simulink model "testing"  (R2013b)
settings: Solver=ode45  StartTime=0.0  StopTime=10.0  RelTol=1e-3
undefined symbols (not defined in the file or in its folder): xlfda_numerator, xlipgetpartsetting
libraries: xbsIndex_r4 x1880, casper_library_delays x19, dspsigops x16, casper_library_misc x8, simulink x1, xps_library x1
(part 10 of 17)

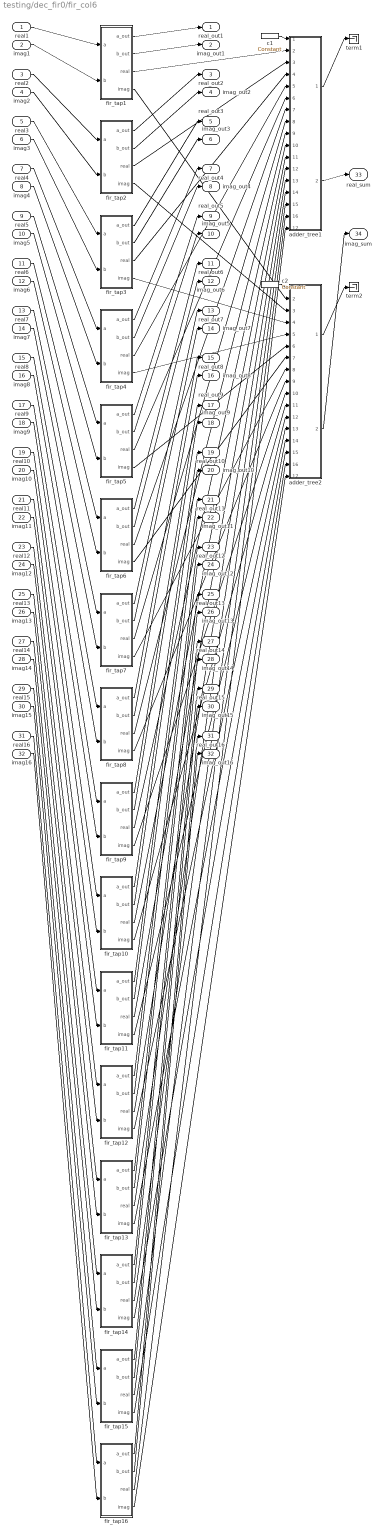
== system testing/dec_fir0/fir_col6 ==
  real1 : Inport
  imag1 : Inport  Port=2
  real2 : Inport  Port=3
  imag2 : Inport  Port=4
  real3 : Inport  Port=5
  imag3 : Inport  Port=6
  real4 : Inport  Port=7
  imag4 : Inport  Port=8
  real5 : Inport  Port=9
  imag5 : Inport  Port=10
  real6 : Inport  Port=11
  imag6 : Inport  Port=12
  real7 : Inport  Port=13
  imag7 : Inport  Port=14
  real8 : Inport  Port=15
  imag8 : Inport  Port=16
  real9 : Inport  Port=17
  imag9 : Inport  Port=18
  real10 : Inport  Port=19
  imag10 : Inport  Port=20
  real11 : Inport  Port=21
  imag11 : Inport  Port=22
  real12 : Inport  Port=23
  imag12 : Inport  Port=24
  real13 : Inport  Port=25
  imag13 : Inport  Port=26
  real14 : Inport  Port=27
  imag14 : Inport  Port=28
  real15 : Inport  Port=29
  imag15 : Inport  Port=30
  real16 : Inport  Port=31
  imag16 : Inport  Port=32
  adder_tree1 : Subsystem  AncestorBlock=casper_library_misc/adder_tree  mask(adder_tree){n_inputs=16, latency=1, adder_imp=DSP48, first_stage_hdl=on}
      mask prompts: n_inputs "Number of Inputs"; latency "Add Latency"; adder_imp "Adder implementation"; first_stage_hdl "Use behavioural HDL for first stage of adders"
      mask help:
      | Sums all inputs using a tree of adds and delays.
      |
      | Number of inputs: The number of inputs to the block to be summed
      | Add latency: The number of clock cycles to perform one addition (affects timing)..
      | Adder implementation: choice of fabric or DSP48E core, or behavioral HDL
      | Use behavioural HDL for first stage of adders: Causes the first stage of adders to be absorbed into DSP blocks if multipliers precede them (Virtex 5). Overrides Adder implementation
      mask init:
      | adder_tree_init(gcb, ...
      |     'n_inputs', n_inputs, ...
      |     'latency', latency, ...
      |     'adder_imp', adder_imp, ...
      |     'first_stage_hdl', first_stage_hdl);
      settings: AttributesFormatString=latency 4
      mask Help: eval('xlWeb(''http://casper.berkeley.edu/wiki/Adder_tree'')')
      mask TypeOptions adder_imp: Behavioral | Fabric | DSP48
  adder_tree2 : Subsystem  AncestorBlock=casper_library_misc/adder_tree  mask(adder_tree){n_inputs=16, latency=1, adder_imp=DSP48, first_stage_hdl=on}
      mask prompts: n_inputs "Number of Inputs"; latency "Add Latency"; adder_imp "Adder implementation"; first_stage_hdl "Use behavioural HDL for first stage of adders"
      mask help:
      | Sums all inputs using a tree of adds and delays.
      |
      | Number of inputs: The number of inputs to the block to be summed
      | Add latency: The number of clock cycles to perform one addition (affects timing)..
      | Adder implementation: choice of fabric or DSP48E core, or behavioral HDL
      | Use behavioural HDL for first stage of adders: Causes the first stage of adders to be absorbed into DSP blocks if multipliers precede them (Virtex 5). Overrides Adder implementation
      mask init:
      | adder_tree_init(gcb, ...
      |     'n_inputs', n_inputs, ...
      |     'latency', latency, ...
      |     'adder_imp', adder_imp, ...
      |     'first_stage_hdl', first_stage_hdl);
      settings: AttributesFormatString=latency 4
      mask Help: eval('xlWeb(''http://casper.berkeley.edu/wiki/Adder_tree'')')
      mask TypeOptions adder_imp: Behavioral | Fabric | DSP48
  c1 : xbsIndex_r4/Constant  const=1  gui_display_data_type=Fixed-point  arith_type=Signed (2's comp)  n_bits=16  bin_pt=14  preci_type=Single  exp_width=8  frac_width=24  explicit_period=on  period=1  equ=P=C  opselect=C  inp2=PCIN>>17  opr=+  inp1=P  carry=CIN  dbl_ovrd=off  block_type=constant
  c2 : xbsIndex_r4/Constant  const=1  gui_display_data_type=Fixed-point  arith_type=Signed (2's comp)  n_bits=16  bin_pt=14  preci_type=Single  exp_width=8  frac_width=24  explicit_period=on  period=1  equ=P=C  opselect=C  inp2=PCIN>>17  opr=+  inp1=P  carry=CIN  dbl_ovrd=off  block_type=constant
  fir_tap1 : Subsystem  AncestorBlock=casper_library_downconverter/fir_tap  mask(fir_tap){factor=0.0068851, latency=2, coeff_bit_width=25, coeff_bin_pt=24}
      mask prompts: latency "Mult latency"; coeff_bit_width "Coefficient bit width"; coeff_bin_pt "Coefficient binary point"
      mask help: Multiplies input data with factor specified.
      mask init:
      | fir_tap_init(gcb, ...
      |     'factor', factor, ...
      |     'latency', latency, ...
      |     'coeff_bit_width', coeff_bit_width, ...
      |     'coeff_bin_pt', coeff_bin_pt);
      mask Help: eval('xlWeb(''http://casper.berkeley.edu/wiki/Fir_tap'')')
  fir_tap10 : Subsystem  AncestorBlock=casper_library_downconverter/fir_tap  mask(fir_tap){factor=-0.00040564, latency=2, coeff_bit_width=25, coeff_bin_pt=24}
      mask prompts: latency "Mult latency"; coeff_bit_width "Coefficient bit width"; coeff_bin_pt "Coefficient binary point"
      mask help: Multiplies input data with factor specified.
      mask init:
      | fir_tap_init(gcb, ...
      |     'factor', factor, ...
      |     'latency', latency, ...
      |     'coeff_bit_width', coeff_bit_width, ...
      |     'coeff_bin_pt', coeff_bin_pt);
      mask Help: eval('xlWeb(''http://casper.berkeley.edu/wiki/Fir_tap'')')
  fir_tap11 : Subsystem  AncestorBlock=casper_library_downconverter/fir_tap  mask(fir_tap){factor=-0.002452, latency=2, coeff_bit_width=25, coeff_bin_pt=24}
      mask prompts: latency "Mult latency"; coeff_bit_width "Coefficient bit width"; coeff_bin_pt "Coefficient binary point"
      mask help: Multiplies input data with factor specified.
      mask init:
      | fir_tap_init(gcb, ...
      |     'factor', factor, ...
      |     'latency', latency, ...
      |     'coeff_bit_width', coeff_bit_width, ...
      |     'coeff_bin_pt', coeff_bin_pt);
      mask Help: eval('xlWeb(''http://casper.berkeley.edu/wiki/Fir_tap'')')
  fir_tap12 : Subsystem  AncestorBlock=casper_library_downconverter/fir_tap  mask(fir_tap){factor=-0.0045559, latency=2, coeff_bit_width=25, coeff_bin_pt=24}
      mask prompts: latency "Mult latency"; coeff_bit_width "Coefficient bit width"; coeff_bin_pt "Coefficient binary point"
      mask help: Multiplies input data with factor specified.
      mask init:
      | fir_tap_init(gcb, ...
      |     'factor', factor, ...
      |     'latency', latency, ...
      |     'coeff_bit_width', coeff_bit_width, ...
      |     'coeff_bin_pt', coeff_bin_pt);
      mask Help: eval('xlWeb(''http://casper.berkeley.edu/wiki/Fir_tap'')')
  fir_tap13 : Subsystem  AncestorBlock=casper_library_downconverter/fir_tap  mask(fir_tap){factor=-0.0066339, latency=2, coeff_bit_width=25, coeff_bin_pt=24}
      mask prompts: latency "Mult latency"; coeff_bit_width "Coefficient bit width"; coeff_bin_pt "Coefficient binary point"
      mask help: Multiplies input data with factor specified.
      mask init:
      | fir_tap_init(gcb, ...
      |     'factor', factor, ...
      |     'latency', latency, ...
      |     'coeff_bit_width', coeff_bit_width, ...
      |     'coeff_bin_pt', coeff_bin_pt);
      mask Help: eval('xlWeb(''http://casper.berkeley.edu/wiki/Fir_tap'')')
  fir_tap14 : Subsystem  AncestorBlock=casper_library_downconverter/fir_tap  mask(fir_tap){factor=-0.0085971, latency=2, coeff_bit_width=25, coeff_bin_pt=24}
      mask prompts: latency "Mult latency"; coeff_bit_width "Coefficient bit width"; coeff_bin_pt "Coefficient binary point"
      mask help: Multiplies input data with factor specified.
      mask init:
      | fir_tap_init(gcb, ...
      |     'factor', factor, ...
      |     'latency', latency, ...
      |     'coeff_bit_width', coeff_bit_width, ...
      |     'coeff_bin_pt', coeff_bin_pt);
      mask Help: eval('xlWeb(''http://casper.berkeley.edu/wiki/Fir_tap'')')
  fir_tap15 : Subsystem  AncestorBlock=casper_library_downconverter/fir_tap  mask(fir_tap){factor=-0.010354, latency=2, coeff_bit_width=25, coeff_bin_pt=24}
      mask prompts: latency "Mult latency"; coeff_bit_width "Coefficient bit width"; coeff_bin_pt "Coefficient binary point"
      mask help: Multiplies input data with factor specified.
      mask init:
      | fir_tap_init(gcb, ...
      |     'factor', factor, ...
      |     'latency', latency, ...
      |     'coeff_bit_width', coeff_bit_width, ...
      |     'coeff_bin_pt', coeff_bin_pt);
      mask Help: eval('xlWeb(''http://casper.berkeley.edu/wiki/Fir_tap'')')
  fir_tap16 : Subsystem  AncestorBlock=casper_library_downconverter/fir_tap  mask(fir_tap){factor=-0.011813, latency=2, coeff_bit_width=25, coeff_bin_pt=24}
      mask prompts: latency "Mult latency"; coeff_bit_width "Coefficient bit width"; coeff_bin_pt "Coefficient binary point"
      mask help: Multiplies input data with factor specified.
      mask init:
      | fir_tap_init(gcb, ...
      |     'factor', factor, ...
      |     'latency', latency, ...
      |     'coeff_bit_width', coeff_bit_width, ...
      |     'coeff_bin_pt', coeff_bin_pt);
      mask Help: eval('xlWeb(''http://casper.berkeley.edu/wiki/Fir_tap'')')
  fir_tap2 : Subsystem  AncestorBlock=casper_library_downconverter/fir_tap  mask(fir_tap){factor=0.007301, latency=2, coeff_bit_width=25, coeff_bin_pt=24}
      mask prompts: latency "Mult latency"; coeff_bit_width "Coefficient bit width"; coeff_bin_pt "Coefficient binary point"
      mask help: Multiplies input data with factor specified.
      mask init:
      | fir_tap_init(gcb, ...
      |     'factor', factor, ...
      |     'latency', latency, ...
      |     'coeff_bit_width', coeff_bit_width, ...
      |     'coeff_bin_pt', coeff_bin_pt);
      mask Help: eval('xlWeb(''http://casper.berkeley.edu/wiki/Fir_tap'')')
  fir_tap3 : Subsystem  AncestorBlock=casper_library_downconverter/fir_tap  mask(fir_tap){factor=0.0074255, latency=2, coeff_bit_width=25, coeff_bin_pt=24}
      mask prompts: latency "Mult latency"; coeff_bit_width "Coefficient bit width"; coeff_bin_pt "Coefficient binary point"
      mask help: Multiplies input data with factor specified.
      mask init:
      | fir_tap_init(gcb, ...
      |     'factor', factor, ...
      |     'latency', latency, ...
      |     'coeff_bit_width', coeff_bit_width, ...
      |     'coeff_bin_pt', coeff_bin_pt);
      mask Help: eval('xlWeb(''http://casper.berkeley.edu/wiki/Fir_tap'')')
  fir_tap4 : Subsystem  AncestorBlock=casper_library_downconverter/fir_tap  mask(fir_tap){factor=0.0072334, latency=2, coeff_bit_width=25, coeff_bin_pt=24}
      mask prompts: latency "Mult latency"; coeff_bit_width "Coefficient bit width"; coeff_bin_pt "Coefficient binary point"
      mask help: Multiplies input data with factor specified.
      mask init:
      | fir_tap_init(gcb, ...
      |     'factor', factor, ...
      |     'latency', latency, ...
      |     'coeff_bit_width', coeff_bit_width, ...
      |     'coeff_bin_pt', coeff_bin_pt);
      mask Help: eval('xlWeb(''http://casper.berkeley.edu/wiki/Fir_tap'')')
  fir_tap5 : Subsystem  AncestorBlock=casper_library_downconverter/fir_tap  mask(fir_tap){factor=0.0067112, latency=2, coeff_bit_width=25, coeff_bin_pt=24}
      mask prompts: latency "Mult latency"; coeff_bit_width "Coefficient bit width"; coeff_bin_pt "Coefficient binary point"
      mask help: Multiplies input data with factor specified.
      mask init:
      | fir_tap_init(gcb, ...
      |     'factor', factor, ...
      |     'latency', latency, ...
      |     'coeff_bit_width', coeff_bit_width, ...
      |     'coeff_bin_pt', coeff_bin_pt);
      mask Help: eval('xlWeb(''http://casper.berkeley.edu/wiki/Fir_tap'')')
  fir_tap6 : Subsystem  AncestorBlock=casper_library_downconverter/fir_tap  mask(fir_tap){factor=0.005858, latency=2, coeff_bit_width=25, coeff_bin_pt=24}
      mask prompts: latency "Mult latency"; coeff_bit_width "Coefficient bit width"; coeff_bin_pt "Coefficient binary point"
      mask help: Multiplies input data with factor specified.
      mask init:
      | fir_tap_init(gcb, ...
      |     'factor', factor, ...
      |     'latency', latency, ...
      |     'coeff_bit_width', coeff_bit_width, ...
      |     'coeff_bin_pt', coeff_bin_pt);
      mask Help: eval('xlWeb(''http://casper.berkeley.edu/wiki/Fir_tap'')')
  fir_tap7 : Subsystem  AncestorBlock=casper_library_downconverter/fir_tap  mask(fir_tap){factor=0.0046863, latency=2, coeff_bit_width=25, coeff_bin_pt=24}
      mask prompts: latency "Mult latency"; coeff_bit_width "Coefficient bit width"; coeff_bin_pt "Coefficient binary point"
      mask help: Multiplies input data with factor specified.
      mask init:
      | fir_tap_init(gcb, ...
      |     'factor', factor, ...
      |     'latency', latency, ...
      |     'coeff_bit_width', coeff_bit_width, ...
      |     'coeff_bin_pt', coeff_bin_pt);
      mask Help: eval('xlWeb(''http://casper.berkeley.edu/wiki/Fir_tap'')')
  fir_tap8 : Subsystem  AncestorBlock=casper_library_downconverter/fir_tap  mask(fir_tap){factor=0.0032228, latency=2, coeff_bit_width=25, coeff_bin_pt=24}
      mask prompts: latency "Mult latency"; coeff_bit_width "Coefficient bit width"; coeff_bin_pt "Coefficient binary point"
      mask help: Multiplies input data with factor specified.
      mask init:
      | fir_tap_init(gcb, ...
      |     'factor', factor, ...
      |     'latency', latency, ...
      |     'coeff_bit_width', coeff_bit_width, ...
      |     'coeff_bin_pt', coeff_bin_pt);
      mask Help: eval('xlWeb(''http://casper.berkeley.edu/wiki/Fir_tap'')')
  fir_tap9 : Subsystem  AncestorBlock=casper_library_downconverter/fir_tap  mask(fir_tap){factor=0.0015077, latency=2, coeff_bit_width=25, coeff_bin_pt=24}
      mask prompts: latency "Mult latency"; coeff_bit_width "Coefficient bit width"; coeff_bin_pt "Coefficient binary point"
      mask help: Multiplies input data with factor specified.
      mask init:
      | fir_tap_init(gcb, ...
      |     'factor', factor, ...
      |     'latency', latency, ...
      |     'coeff_bit_width', coeff_bit_width, ...
      |     'coeff_bin_pt', coeff_bin_pt);
      mask Help: eval('xlWeb(''http://casper.berkeley.edu/wiki/Fir_tap'')')
  term1 : Terminator
  term2 : Terminator
  real_out1 : Outport
  imag_out1 : Outport  Port=2
  real_out2 : Outport  Port=3
  imag_out2 : Outport  Port=4
  real_out3 : Outport  Port=5
  imag_out3 : Outport  Port=6
  real_out4 : Outport  Port=7
  imag_out4 : Outport  Port=8
  real_out5 : Outport  Port=9
  imag_out5 : Outport  Port=10
  real_out6 : Outport  Port=11
  imag_out6 : Outport  Port=12
  real_out7 : Outport  Port=13
  imag_out7 : Outport  Port=14
  real_out8 : Outport  Port=15
  imag_out8 : Outport  Port=16
  real_out9 : Outport  Port=17
  imag_out9 : Outport  Port=18
  real_out10 : Outport  Port=19
  imag_out10 : Outport  Port=20
  real_out11 : Outport  Port=21
  imag_out11 : Outport  Port=22
  real_out12 : Outport  Port=23
  imag_out12 : Outport  Port=24
  real_out13 : Outport  Port=25
  imag_out13 : Outport  Port=26
  real_out14 : Outport  Port=27
  imag_out14 : Outport  Port=28
  real_out15 : Outport  Port=29
  imag_out15 : Outport  Port=30
  real_out16 : Outport  Port=31
  imag_out16 : Outport  Port=32
  real_sum : Outport  Port=33
  imag_sum : Outport  Port=34
  wires:
  adder_tree1/1(sync_out) -> term1/1
  adder_tree2/1(sync_out) -> term2/1
  c1/1 -> adder_tree1/1(sync)
  c2/1 -> adder_tree2/1(sync)
  adder_tree1/2(dout) -> real_sum/1
  adder_tree2/2(dout) -> imag_sum/1
  real1/1 -> fir_tap1/1(a)
  imag1/1 -> fir_tap1/2(b)
  fir_tap1/1(a_out) -> real_out1/1
  fir_tap1/2(b_out) -> imag_out1/1
  fir_tap1/3(real) -> adder_tree1/2(din1)
  fir_tap1/4(imag) -> adder_tree2/2(din1)
  real2/1 -> fir_tap2/1(a)
  imag2/1 -> fir_tap2/2(b)
  fir_tap2/1(a_out) -> real_out2/1
  fir_tap2/2(b_out) -> imag_out2/1
  fir_tap2/3(real) -> adder_tree1/3(din2)
  fir_tap2/4(imag) -> adder_tree2/3(din2)
  real3/1 -> fir_tap3/1(a)
  imag3/1 -> fir_tap3/2(b)
  fir_tap3/1(a_out) -> real_out3/1
  fir_tap3/2(b_out) -> imag_out3/1
  fir_tap3/3(real) -> adder_tree1/4(din3)
  fir_tap3/4(imag) -> adder_tree2/4(din3)
  real4/1 -> fir_tap4/1(a)
  imag4/1 -> fir_tap4/2(b)
  fir_tap4/1(a_out) -> real_out4/1
  fir_tap4/2(b_out) -> imag_out4/1
  fir_tap4/3(real) -> adder_tree1/5(din4)
  fir_tap4/4(imag) -> adder_tree2/5(din4)
  real5/1 -> fir_tap5/1(a)
  imag5/1 -> fir_tap5/2(b)
  fir_tap5/1(a_out) -> real_out5/1
  fir_tap5/2(b_out) -> imag_out5/1
  fir_tap5/3(real) -> adder_tree1/6(din5)
  fir_tap5/4(imag) -> adder_tree2/6(din5)
  real6/1 -> fir_tap6/1(a)
  imag6/1 -> fir_tap6/2(b)
  fir_tap6/1(a_out) -> real_out6/1
  fir_tap6/2(b_out) -> imag_out6/1
  fir_tap6/3(real) -> adder_tree1/7(din6)
  fir_tap6/4(imag) -> adder_tree2/7(din6)
  real7/1 -> fir_tap7/1(a)
  imag7/1 -> fir_tap7/2(b)
  fir_tap7/1(a_out) -> real_out7/1
  fir_tap7/2(b_out) -> imag_out7/1
  fir_tap7/3(real) -> adder_tree1/8(din7)
  fir_tap7/4(imag) -> adder_tree2/8(din7)
  real8/1 -> fir_tap8/1(a)
  imag8/1 -> fir_tap8/2(b)
  fir_tap8/1(a_out) -> real_out8/1
  fir_tap8/2(b_out) -> imag_out8/1
  fir_tap8/3(real) -> adder_tree1/9(din8)
  fir_tap8/4(imag) -> adder_tree2/9(din8)
  real9/1 -> fir_tap9/1(a)
  imag9/1 -> fir_tap9/2(b)
  fir_tap9/1(a_out) -> real_out9/1
  fir_tap9/2(b_out) -> imag_out9/1
  fir_tap9/3(real) -> adder_tree1/10(din9)
  fir_tap9/4(imag) -> adder_tree2/10(din9)
  real10/1 -> fir_tap10/1(a)
  imag10/1 -> fir_tap10/2(b)
  fir_tap10/1(a_out) -> real_out10/1
  fir_tap10/2(b_out) -> imag_out10/1
  fir_tap10/3(real) -> adder_tree1/11(din10)
  fir_tap10/4(imag) -> adder_tree2/11(din10)
  real11/1 -> fir_tap11/1(a)
  imag11/1 -> fir_tap11/2(b)
  fir_tap11/1(a_out) -> real_out11/1
  fir_tap11/2(b_out) -> imag_out11/1
  fir_tap11/3(real) -> adder_tree1/12(din11)
  fir_tap11/4(imag) -> adder_tree2/12(din11)
  real12/1 -> fir_tap12/1(a)
  imag12/1 -> fir_tap12/2(b)
  fir_tap12/1(a_out) -> real_out12/1
  fir_tap12/2(b_out) -> imag_out12/1
  fir_tap12/3(real) -> adder_tree1/13(din12)
  fir_tap12/4(imag) -> adder_tree2/13(din12)
  real13/1 -> fir_tap13/1(a)
  imag13/1 -> fir_tap13/2(b)
  fir_tap13/1(a_out) -> real_out13/1
  fir_tap13/2(b_out) -> imag_out13/1
  fir_tap13/3(real) -> adder_tree1/14(din13)
  fir_tap13/4(imag) -> adder_tree2/14(din13)
  real14/1 -> fir_tap14/1(a)
  imag14/1 -> fir_tap14/2(b)
  fir_tap14/1(a_out) -> real_out14/1
  fir_tap14/2(b_out) -> imag_out14/1
  fir_tap14/3(real) -> adder_tree1/15(din14)
  fir_tap14/4(imag) -> adder_tree2/15(din14)
  real15/1 -> fir_tap15/1(a)
  imag15/1 -> fir_tap15/2(b)
  fir_tap15/1(a_out) -> real_out15/1
  fir_tap15/2(b_out) -> imag_out15/1
  fir_tap15/3(real) -> adder_tree1/16(din15)
  fir_tap15/4(imag) -> adder_tree2/16(din15)
  real16/1 -> fir_tap16/1(a)
  imag16/1 -> fir_tap16/2(b)
  fir_tap16/1(a_out) -> real_out16/1
  fir_tap16/2(b_out) -> imag_out16/1
  fir_tap16/3(real) -> adder_tree1/17(din16)
  fir_tap16/4(imag) -> adder_tree2/17(din16)

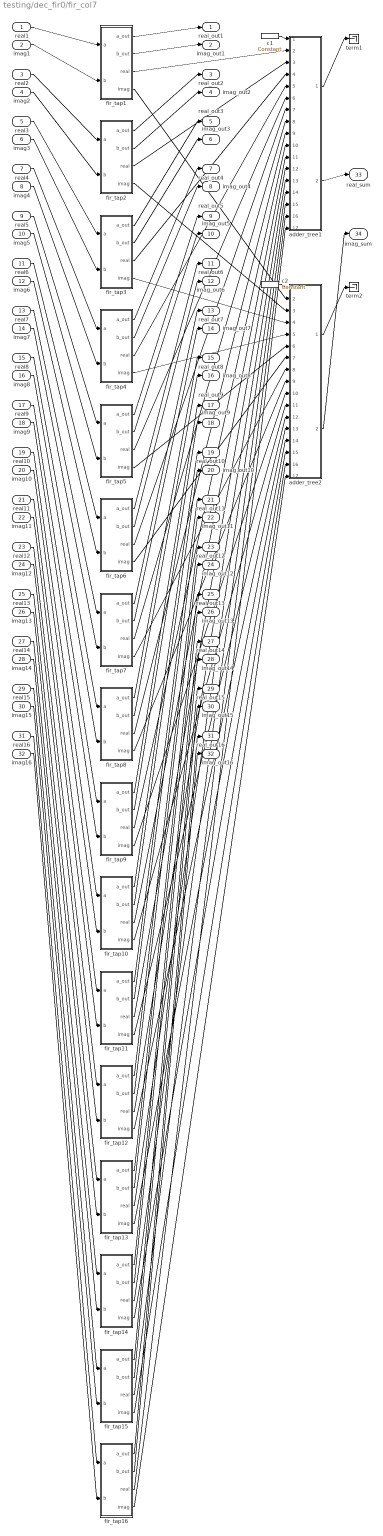
== system testing/dec_fir0/fir_col7 ==
  real1 : Inport
  imag1 : Inport  Port=2
  real2 : Inport  Port=3
  imag2 : Inport  Port=4
  real3 : Inport  Port=5
  imag3 : Inport  Port=6
  real4 : Inport  Port=7
  imag4 : Inport  Port=8
  real5 : Inport  Port=9
  imag5 : Inport  Port=10
  real6 : Inport  Port=11
  imag6 : Inport  Port=12
  real7 : Inport  Port=13
  imag7 : Inport  Port=14
  real8 : Inport  Port=15
  imag8 : Inport  Port=16
  real9 : Inport  Port=17
  imag9 : Inport  Port=18
  real10 : Inport  Port=19
  imag10 : Inport  Port=20
  real11 : Inport  Port=21
  imag11 : Inport  Port=22
  real12 : Inport  Port=23
  imag12 : Inport  Port=24
  real13 : Inport  Port=25
  imag13 : Inport  Port=26
  real14 : Inport  Port=27
  imag14 : Inport  Port=28
  real15 : Inport  Port=29
  imag15 : Inport  Port=30
  real16 : Inport  Port=31
  imag16 : Inport  Port=32
  adder_tree1 : Subsystem  AncestorBlock=casper_library_misc/adder_tree  mask(adder_tree){n_inputs=16, latency=1, adder_imp=DSP48, first_stage_hdl=on}
      mask prompts: n_inputs "Number of Inputs"; latency "Add Latency"; adder_imp "Adder implementation"; first_stage_hdl "Use behavioural HDL for first stage of adders"
      mask help:
      | Sums all inputs using a tree of adds and delays.
      |
      | Number of inputs: The number of inputs to the block to be summed
      | Add latency: The number of clock cycles to perform one addition (affects timing)..
      | Adder implementation: choice of fabric or DSP48E core, or behavioral HDL
      | Use behavioural HDL for first stage of adders: Causes the first stage of adders to be absorbed into DSP blocks if multipliers precede them (Virtex 5). Overrides Adder implementation
      mask init:
      | adder_tree_init(gcb, ...
      |     'n_inputs', n_inputs, ...
      |     'latency', latency, ...
      |     'adder_imp', adder_imp, ...
      |     'first_stage_hdl', first_stage_hdl);
      settings: AttributesFormatString=latency 4
      mask Help: eval('xlWeb(''http://casper.berkeley.edu/wiki/Adder_tree'')')
      mask TypeOptions adder_imp: Behavioral | Fabric | DSP48
  adder_tree2 : Subsystem  AncestorBlock=casper_library_misc/adder_tree  mask(adder_tree){n_inputs=16, latency=1, adder_imp=DSP48, first_stage_hdl=on}
      mask prompts: n_inputs "Number of Inputs"; latency "Add Latency"; adder_imp "Adder implementation"; first_stage_hdl "Use behavioural HDL for first stage of adders"
      mask help:
      | Sums all inputs using a tree of adds and delays.
      |
      | Number of inputs: The number of inputs to the block to be summed
      | Add latency: The number of clock cycles to perform one addition (affects timing)..
      | Adder implementation: choice of fabric or DSP48E core, or behavioral HDL
      | Use behavioural HDL for first stage of adders: Causes the first stage of adders to be absorbed into DSP blocks if multipliers precede them (Virtex 5). Overrides Adder implementation
      mask init:
      | adder_tree_init(gcb, ...
      |     'n_inputs', n_inputs, ...
      |     'latency', latency, ...
      |     'adder_imp', adder_imp, ...
      |     'first_stage_hdl', first_stage_hdl);
      settings: AttributesFormatString=latency 4
      mask Help: eval('xlWeb(''http://casper.berkeley.edu/wiki/Adder_tree'')')
      mask TypeOptions adder_imp: Behavioral | Fabric | DSP48
  c1 : xbsIndex_r4/Constant  const=1  gui_display_data_type=Fixed-point  arith_type=Signed (2's comp)  n_bits=16  bin_pt=14  preci_type=Single  exp_width=8  frac_width=24  explicit_period=on  period=1  equ=P=C  opselect=C  inp2=PCIN>>17  opr=+  inp1=P  carry=CIN  dbl_ovrd=off  block_type=constant
  c2 : xbsIndex_r4/Constant  const=1  gui_display_data_type=Fixed-point  arith_type=Signed (2's comp)  n_bits=16  bin_pt=14  preci_type=Single  exp_width=8  frac_width=24  explicit_period=on  period=1  equ=P=C  opselect=C  inp2=PCIN>>17  opr=+  inp1=P  carry=CIN  dbl_ovrd=off  block_type=constant
  fir_tap1 : Subsystem  AncestorBlock=casper_library_downconverter/fir_tap  mask(fir_tap){factor=-0.0040983, latency=2, coeff_bit_width=25, coeff_bin_pt=24}
      mask prompts: latency "Mult latency"; coeff_bit_width "Coefficient bit width"; coeff_bin_pt "Coefficient binary point"
      mask help: Multiplies input data with factor specified.
      mask init:
      | fir_tap_init(gcb, ...
      |     'factor', factor, ...
      |     'latency', latency, ...
      |     'coeff_bit_width', coeff_bit_width, ...
      |     'coeff_bin_pt', coeff_bin_pt);
      mask Help: eval('xlWeb(''http://casper.berkeley.edu/wiki/Fir_tap'')')
  fir_tap10 : Subsystem  AncestorBlock=casper_library_downconverter/fir_tap  mask(fir_tap){factor=-0.00052147, latency=2, coeff_bit_width=25, coeff_bin_pt=24}
      mask prompts: latency "Mult latency"; coeff_bit_width "Coefficient bit width"; coeff_bin_pt "Coefficient binary point"
      mask help: Multiplies input data with factor specified.
      mask init:
      | fir_tap_init(gcb, ...
      |     'factor', factor, ...
      |     'latency', latency, ...
      |     'coeff_bit_width', coeff_bit_width, ...
      |     'coeff_bin_pt', coeff_bin_pt);
      mask Help: eval('xlWeb(''http://casper.berkeley.edu/wiki/Fir_tap'')')
  fir_tap11 : Subsystem  AncestorBlock=casper_library_downconverter/fir_tap  mask(fir_tap){factor=0.00066203, latency=2, coeff_bit_width=25, coeff_bin_pt=24}
      mask prompts: latency "Mult latency"; coeff_bit_width "Coefficient bit width"; coeff_bin_pt "Coefficient binary point"
      mask help: Multiplies input data with factor specified.
      mask init:
      | fir_tap_init(gcb, ...
      |     'factor', factor, ...
      |     'latency', latency, ...
      |     'coeff_bit_width', coeff_bit_width, ...
      |     'coeff_bin_pt', coeff_bin_pt);
      mask Help: eval('xlWeb(''http://casper.berkeley.edu/wiki/Fir_tap'')')
  fir_tap12 : Subsystem  AncestorBlock=casper_library_downconverter/fir_tap  mask(fir_tap){factor=0.00189, latency=2, coeff_bit_width=25, coeff_bin_pt=24}
      mask prompts: latency "Mult latency"; coeff_bit_width "Coefficient bit width"; coeff_bin_pt "Coefficient binary point"
      mask help: Multiplies input data with factor specified.
      mask init:
      | fir_tap_init(gcb, ...
      |     'factor', factor, ...
      |     'latency', latency, ...
      |     'coeff_bit_width', coeff_bit_width, ...
      |     'coeff_bin_pt', coeff_bin_pt);
      mask Help: eval('xlWeb(''http://casper.berkeley.edu/wiki/Fir_tap'')')
  fir_tap13 : Subsystem  AncestorBlock=casper_library_downconverter/fir_tap  mask(fir_tap){factor=0.0031122, latency=2, coeff_bit_width=25, coeff_bin_pt=24}
      mask prompts: latency "Mult latency"; coeff_bit_width "Coefficient bit width"; coeff_bin_pt "Coefficient binary point"
      mask help: Multiplies input data with factor specified.
      mask init:
      | fir_tap_init(gcb, ...
      |     'factor', factor, ...
      |     'latency', latency, ...
      |     'coeff_bit_width', coeff_bit_width, ...
      |     'coeff_bin_pt', coeff_bin_pt);
      mask Help: eval('xlWeb(''http://casper.berkeley.edu/wiki/Fir_tap'')')
  fir_tap14 : Subsystem  AncestorBlock=casper_library_downconverter/fir_tap  mask(fir_tap){factor=0.0042757, latency=2, coeff_bit_width=25, coeff_bin_pt=24}
      mask prompts: latency "Mult latency"; coeff_bit_width "Coefficient bit width"; coeff_bin_pt "Coefficient binary point"
      mask help: Multiplies input data with factor specified.
      mask init:
      | fir_tap_init(gcb, ...
      |     'factor', factor, ...
      |     'latency', latency, ...
      |     'coeff_bit_width', coeff_bit_width, ...
      |     'coeff_bin_pt', coeff_bin_pt);
      mask Help: eval('xlWeb(''http://casper.berkeley.edu/wiki/Fir_tap'')')
  fir_tap15 : Subsystem  AncestorBlock=casper_library_downconverter/fir_tap  mask(fir_tap){factor=0.0053266, latency=2, coeff_bit_width=25, coeff_bin_pt=24}
      mask prompts: latency "Mult latency"; coeff_bit_width "Coefficient bit width"; coeff_bin_pt "Coefficient binary point"
      mask help: Multiplies input data with factor specified.
      mask init:
      | fir_tap_init(gcb, ...
      |     'factor', factor, ...
      |     'latency', latency, ...
      |     'coeff_bit_width', coeff_bit_width, ...
      |     'coeff_bin_pt', coeff_bin_pt);
      mask Help: eval('xlWeb(''http://casper.berkeley.edu/wiki/Fir_tap'')')
  fir_tap16 : Subsystem  AncestorBlock=casper_library_downconverter/fir_tap  mask(fir_tap){factor=0.0062127, latency=2, coeff_bit_width=25, coeff_bin_pt=24}
      mask prompts: latency "Mult latency"; coeff_bit_width "Coefficient bit width"; coeff_bin_pt "Coefficient binary point"
      mask help: Multiplies input data with factor specified.
      mask init:
      | fir_tap_init(gcb, ...
      |     'factor', factor, ...
      |     'latency', latency, ...
      |     'coeff_bit_width', coeff_bit_width, ...
      |     'coeff_bin_pt', coeff_bin_pt);
      mask Help: eval('xlWeb(''http://casper.berkeley.edu/wiki/Fir_tap'')')
  fir_tap2 : Subsystem  AncestorBlock=casper_library_downconverter/fir_tap  mask(fir_tap){factor=-0.0044554, latency=2, coeff_bit_width=25, coeff_bin_pt=24}
      mask prompts: latency "Mult latency"; coeff_bit_width "Coefficient bit width"; coeff_bin_pt "Coefficient binary point"
      mask help: Multiplies input data with factor specified.
      mask init:
      | fir_tap_init(gcb, ...
      |     'factor', factor, ...
      |     'latency', latency, ...
      |     'coeff_bit_width', coeff_bit_width, ...
      |     'coeff_bin_pt', coeff_bin_pt);
      mask Help: eval('xlWeb(''http://casper.berkeley.edu/wiki/Fir_tap'')')
  fir_tap3 : Subsystem  AncestorBlock=casper_library_downconverter/fir_tap  mask(fir_tap){factor=-0.0046386, latency=2, coeff_bit_width=25, coeff_bin_pt=24}
      mask prompts: latency "Mult latency"; coeff_bit_width "Coefficient bit width"; coeff_bin_pt "Coefficient binary point"
      mask help: Multiplies input data with factor specified.
      mask init:
      | fir_tap_init(gcb, ...
      |     'factor', factor, ...
      |     'latency', latency, ...
      |     'coeff_bit_width', coeff_bit_width, ...
      |     'coeff_bin_pt', coeff_bin_pt);
      mask Help: eval('xlWeb(''http://casper.berkeley.edu/wiki/Fir_tap'')')
  fir_tap4 : Subsystem  AncestorBlock=casper_library_downconverter/fir_tap  mask(fir_tap){factor=-0.0046295, latency=2, coeff_bit_width=25, coeff_bin_pt=24}
      mask prompts: latency "Mult latency"; coeff_bit_width "Coefficient bit width"; coeff_bin_pt "Coefficient binary point"
      mask help: Multiplies input data with factor specified.
      mask init:
      | fir_tap_init(gcb, ...
      |     'factor', factor, ...
      |     'latency', latency, ...
      |     'coeff_bit_width', coeff_bit_width, ...
      |     'coeff_bin_pt', coeff_bin_pt);
      mask Help: eval('xlWeb(''http://casper.berkeley.edu/wiki/Fir_tap'')')
  fir_tap5 : Subsystem  AncestorBlock=casper_library_downconverter/fir_tap  mask(fir_tap){factor=-0.0044174, latency=2, coeff_bit_width=25, coeff_bin_pt=24}
      mask prompts: latency "Mult latency"; coeff_bit_width "Coefficient bit width"; coeff_bin_pt "Coefficient binary point"
      mask help: Multiplies input data with factor specified.
      mask init:
      | fir_tap_init(gcb, ...
      |     'factor', factor, ...
      |     'latency', latency, ...
      |     'coeff_bit_width', coeff_bit_width, ...
      |     'coeff_bin_pt', coeff_bin_pt);
      mask Help: eval('xlWeb(''http://casper.berkeley.edu/wiki/Fir_tap'')')
  fir_tap6 : Subsystem  AncestorBlock=casper_library_downconverter/fir_tap  mask(fir_tap){factor=-0.0039996, latency=2, coeff_bit_width=25, coeff_bin_pt=24}
      mask prompts: latency "Mult latency"; coeff_bit_width "Coefficient bit width"; coeff_bin_pt "Coefficient binary point"
      mask help: Multiplies input data with factor specified.
      mask init:
      | fir_tap_init(gcb, ...
      |     'factor', factor, ...
      |     'latency', latency, ...
      |     'coeff_bit_width', coeff_bit_width, ...
      |     'coeff_bin_pt', coeff_bin_pt);
      mask Help: eval('xlWeb(''http://casper.berkeley.edu/wiki/Fir_tap'')')
  fir_tap7 : Subsystem  AncestorBlock=casper_library_downconverter/fir_tap  mask(fir_tap){factor=-0.0033818, latency=2, coeff_bit_width=25, coeff_bin_pt=24}
      mask prompts: latency "Mult latency"; coeff_bit_width "Coefficient bit width"; coeff_bin_pt "Coefficient binary point"
      mask help: Multiplies input data with factor specified.
      mask init:
      | fir_tap_init(gcb, ...
      |     'factor', factor, ...
      |     'latency', latency, ...
      |     'coeff_bit_width', coeff_bit_width, ...
      |     'coeff_bin_pt', coeff_bin_pt);
      mask Help: eval('xlWeb(''http://casper.berkeley.edu/wiki/Fir_tap'')')
  fir_tap8 : Subsystem  AncestorBlock=casper_library_downconverter/fir_tap  mask(fir_tap){factor=-0.0025791, latency=2, coeff_bit_width=25, coeff_bin_pt=24}
      mask prompts: latency "Mult latency"; coeff_bit_width "Coefficient bit width"; coeff_bin_pt "Coefficient binary point"
      mask help: Multiplies input data with factor specified.
      mask init:
      | fir_tap_init(gcb, ...
      |     'factor', factor, ...
      |     'latency', latency, ...
      |     'coeff_bit_width', coeff_bit_width, ...
      |     'coeff_bin_pt', coeff_bin_pt);
      mask Help: eval('xlWeb(''http://casper.berkeley.edu/wiki/Fir_tap'')')
  fir_tap9 : Subsystem  AncestorBlock=casper_library_downconverter/fir_tap  mask(fir_tap){factor=-0.001615, latency=2, coeff_bit_width=25, coeff_bin_pt=24}
      mask prompts: latency "Mult latency"; coeff_bit_width "Coefficient bit width"; coeff_bin_pt "Coefficient binary point"
      mask help: Multiplies input data with factor specified.
      mask init:
      | fir_tap_init(gcb, ...
      |     'factor', factor, ...
      |     'latency', latency, ...
      |     'coeff_bit_width', coeff_bit_width, ...
      |     'coeff_bin_pt', coeff_bin_pt);
      mask Help: eval('xlWeb(''http://casper.berkeley.edu/wiki/Fir_tap'')')
  term1 : Terminator
  term2 : Terminator
  real_out1 : Outport
  imag_out1 : Outport  Port=2
  real_out2 : Outport  Port=3
  imag_out2 : Outport  Port=4
  real_out3 : Outport  Port=5
  imag_out3 : Outport  Port=6
  real_out4 : Outport  Port=7
  imag_out4 : Outport  Port=8
  real_out5 : Outport  Port=9
  imag_out5 : Outport  Port=10
  real_out6 : Outport  Port=11
  imag_out6 : Outport  Port=12
  real_out7 : Outport  Port=13
  imag_out7 : Outport  Port=14
  real_out8 : Outport  Port=15
  imag_out8 : Outport  Port=16
  real_out9 : Outport  Port=17
  imag_out9 : Outport  Port=18
  real_out10 : Outport  Port=19
  imag_out10 : Outport  Port=20
  real_out11 : Outport  Port=21
  imag_out11 : Outport  Port=22
  real_out12 : Outport  Port=23
  imag_out12 : Outport  Port=24
  real_out13 : Outport  Port=25
  imag_out13 : Outport  Port=26
  real_out14 : Outport  Port=27
  imag_out14 : Outport  Port=28
  real_out15 : Outport  Port=29
  imag_out15 : Outport  Port=30
  real_out16 : Outport  Port=31
  imag_out16 : Outport  Port=32
  real_sum : Outport  Port=33
  imag_sum : Outport  Port=34
  wires:
  adder_tree1/1(sync_out) -> term1/1
  adder_tree2/1(sync_out) -> term2/1
  c1/1 -> adder_tree1/1(sync)
  c2/1 -> adder_tree2/1(sync)
  adder_tree1/2(dout) -> real_sum/1
  adder_tree2/2(dout) -> imag_sum/1
  real1/1 -> fir_tap1/1(a)
  imag1/1 -> fir_tap1/2(b)
  fir_tap1/1(a_out) -> real_out1/1
  fir_tap1/2(b_out) -> imag_out1/1
  fir_tap1/3(real) -> adder_tree1/2(din1)
  fir_tap1/4(imag) -> adder_tree2/2(din1)
  real2/1 -> fir_tap2/1(a)
  imag2/1 -> fir_tap2/2(b)
  fir_tap2/1(a_out) -> real_out2/1
  fir_tap2/2(b_out) -> imag_out2/1
  fir_tap2/3(real) -> adder_tree1/3(din2)
  fir_tap2/4(imag) -> adder_tree2/3(din2)
  real3/1 -> fir_tap3/1(a)
  imag3/1 -> fir_tap3/2(b)
  fir_tap3/1(a_out) -> real_out3/1
  fir_tap3/2(b_out) -> imag_out3/1
  fir_tap3/3(real) -> adder_tree1/4(din3)
  fir_tap3/4(imag) -> adder_tree2/4(din3)
  real4/1 -> fir_tap4/1(a)
  imag4/1 -> fir_tap4/2(b)
  fir_tap4/1(a_out) -> real_out4/1
  fir_tap4/2(b_out) -> imag_out4/1
  fir_tap4/3(real) -> adder_tree1/5(din4)
  fir_tap4/4(imag) -> adder_tree2/5(din4)
  real5/1 -> fir_tap5/1(a)
  imag5/1 -> fir_tap5/2(b)
  fir_tap5/1(a_out) -> real_out5/1
  fir_tap5/2(b_out) -> imag_out5/1
  fir_tap5/3(real) -> adder_tree1/6(din5)
  fir_tap5/4(imag) -> adder_tree2/6(din5)
  real6/1 -> fir_tap6/1(a)
  imag6/1 -> fir_tap6/2(b)
  fir_tap6/1(a_out) -> real_out6/1
  fir_tap6/2(b_out) -> imag_out6/1
  fir_tap6/3(real) -> adder_tree1/7(din6)
  fir_tap6/4(imag) -> adder_tree2/7(din6)
  real7/1 -> fir_tap7/1(a)
  imag7/1 -> fir_tap7/2(b)
  fir_tap7/1(a_out) -> real_out7/1
  fir_tap7/2(b_out) -> imag_out7/1
  fir_tap7/3(real) -> adder_tree1/8(din7)
  fir_tap7/4(imag) -> adder_tree2/8(din7)
  real8/1 -> fir_tap8/1(a)
  imag8/1 -> fir_tap8/2(b)
  fir_tap8/1(a_out) -> real_out8/1
  fir_tap8/2(b_out) -> imag_out8/1
  fir_tap8/3(real) -> adder_tree1/9(din8)
  fir_tap8/4(imag) -> adder_tree2/9(din8)
  real9/1 -> fir_tap9/1(a)
  imag9/1 -> fir_tap9/2(b)
  fir_tap9/1(a_out) -> real_out9/1
  fir_tap9/2(b_out) -> imag_out9/1
  fir_tap9/3(real) -> adder_tree1/10(din9)
  fir_tap9/4(imag) -> adder_tree2/10(din9)
  real10/1 -> fir_tap10/1(a)
  imag10/1 -> fir_tap10/2(b)
  fir_tap10/1(a_out) -> real_out10/1
  fir_tap10/2(b_out) -> imag_out10/1
  fir_tap10/3(real) -> adder_tree1/11(din10)
  fir_tap10/4(imag) -> adder_tree2/11(din10)
  real11/1 -> fir_tap11/1(a)
  imag11/1 -> fir_tap11/2(b)
  fir_tap11/1(a_out) -> real_out11/1
  fir_tap11/2(b_out) -> imag_out11/1
  fir_tap11/3(real) -> adder_tree1/12(din11)
  fir_tap11/4(imag) -> adder_tree2/12(din11)
  real12/1 -> fir_tap12/1(a)
  imag12/1 -> fir_tap12/2(b)
  fir_tap12/1(a_out) -> real_out12/1
  fir_tap12/2(b_out) -> imag_out12/1
  fir_tap12/3(real) -> adder_tree1/13(din12)
  fir_tap12/4(imag) -> adder_tree2/13(din12)
  real13/1 -> fir_tap13/1(a)
  imag13/1 -> fir_tap13/2(b)
  fir_tap13/1(a_out) -> real_out13/1
  fir_tap13/2(b_out) -> imag_out13/1
  fir_tap13/3(real) -> adder_tree1/14(din13)
  fir_tap13/4(imag) -> adder_tree2/14(din13)
  real14/1 -> fir_tap14/1(a)
  imag14/1 -> fir_tap14/2(b)
  fir_tap14/1(a_out) -> real_out14/1
  fir_tap14/2(b_out) -> imag_out14/1
  fir_tap14/3(real) -> adder_tree1/15(din14)
  fir_tap14/4(imag) -> adder_tree2/15(din14)
  real15/1 -> fir_tap15/1(a)
  imag15/1 -> fir_tap15/2(b)
  fir_tap15/1(a_out) -> real_out15/1
  fir_tap15/2(b_out) -> imag_out15/1
  fir_tap15/3(real) -> adder_tree1/16(din15)
  fir_tap15/4(imag) -> adder_tree2/16(din15)
  real16/1 -> fir_tap16/1(a)
  imag16/1 -> fir_tap16/2(b)
  fir_tap16/1(a_out) -> real_out16/1
  fir_tap16/2(b_out) -> imag_out16/1
  fir_tap16/3(real) -> adder_tree1/17(din16)
  fir_tap16/4(imag) -> adder_tree2/17(din16)

== system testing/dec_fir0/imag_sum ==
  sync : Inport
  din1 : Inport  Port=2
  din2 : Inport  Port=3
  din3 : Inport  Port=4
  din4 : Inport  Port=5
  din5 : Inport  Port=6
  din6 : Inport  Port=7
  din7 : Inport  Port=8
  addr{1..3,5..7} (6 alike) : xbsIndex_r4/AddSub  mode=Addition  use_carryin=off  use_carryout=off  en=off  latency=1  precision=Full  arith_type=Unsigned  n_bits=16  bin_pt=14  quantization=Truncate  overflow=Wrap  dbl_ovrd=off  use_behavioral_HDL=off  hw_selection=DSP48  pipelined=on  use_rpm=on  block_type=addsub
  dly4 : xbsIndex_r4/Delay  rst=off  infoeditControl=Selection of Reset will increase slice count due to use of real FFs and instead of SRLs  en=off  latency=1  dbl_ovrd=off  reg_retiming=on  block_type=delay
  sync_delay : xbsIndex_r4/Delay  rst=off  infoeditControl=Selection of Reset will increase slice count due to use of real FFs and instead of SRLs  en=off  latency=3  dbl_ovrd=off  reg_retiming=on  block_type=delay
      settings: block_version=11.4
  sync_out : Outport
  dout : Outport  Port=2
  wires:
  sync/1 -> sync_delay/1
  sync_delay/1 -> sync_out/1
  din1/1 -> addr1/1
  din2/1 -> addr1/2
  din3/1 -> addr2/1
  din4/1 -> addr2/2
  din5/1 -> addr3/1
  din6/1 -> addr3/2
  din7/1 -> dly4/1
  addr1/1 -> addr5/1
  addr2/1 -> addr5/2
  addr3/1 -> addr6/1
  dly4/1 -> addr6/2
  addr5/1 -> addr7/1
  addr6/1 -> addr7/2
  addr7/1 -> dout/1

== system testing/dec_fir0/real_sum ==
  sync : Inport
  din1 : Inport  Port=2
  din2 : Inport  Port=3
  din3 : Inport  Port=4
  din4 : Inport  Port=5
  din5 : Inport  Port=6
  din6 : Inport  Port=7
  din7 : Inport  Port=8
  addr{1..3,5..7} (6 alike) : xbsIndex_r4/AddSub  mode=Addition  use_carryin=off  use_carryout=off  en=off  latency=1  precision=Full  arith_type=Unsigned  n_bits=16  bin_pt=14  quantization=Truncate  overflow=Wrap  dbl_ovrd=off  use_behavioral_HDL=off  hw_selection=DSP48  pipelined=on  use_rpm=on  block_type=addsub
  dly4 : xbsIndex_r4/Delay  rst=off  infoeditControl=Selection of Reset will increase slice count due to use of real FFs and instead of SRLs  en=off  latency=1  dbl_ovrd=off  reg_retiming=on  block_type=delay
  sync_delay : xbsIndex_r4/Delay  rst=off  infoeditControl=Selection of Reset will increase slice count due to use of real FFs and instead of SRLs  en=off  latency=3  dbl_ovrd=off  reg_retiming=on  block_type=delay
      settings: block_version=11.4
  sync_out : Outport
  dout : Outport  Port=2
  wires:
  sync/1 -> sync_delay/1
  sync_delay/1 -> sync_out/1
  din1/1 -> addr1/1
  din2/1 -> addr1/2
  din3/1 -> addr2/1
  din4/1 -> addr2/2
  din5/1 -> addr3/1
  din6/1 -> addr3/2
  din7/1 -> dly4/1
  addr1/1 -> addr5/1
  addr2/1 -> addr5/2
  addr3/1 -> addr6/1
  dly4/1 -> addr6/2
  addr5/1 -> addr7/1
  addr6/1 -> addr7/2
  addr7/1 -> dout/1

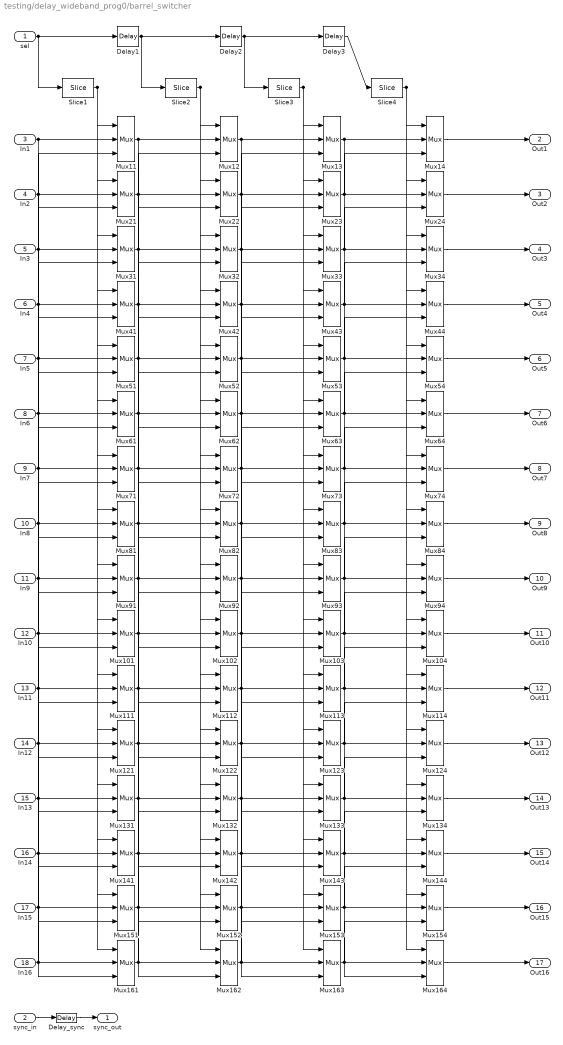
== system testing/delay_wideband_prog0/barrel_switcher ==
  sel : Inport
  sync_in : Inport  Port=2
  In1 : Inport  Port=3
  In2 : Inport  Port=4
  In3 : Inport  Port=5
  In4 : Inport  Port=6
  In5 : Inport  Port=7
  In6 : Inport  Port=8
  In7 : Inport  Port=9
  In8 : Inport  Port=10
  In9 : Inport  Port=11
  In10 : Inport  Port=12
  In11 : Inport  Port=13
  In12 : Inport  Port=14
  In13 : Inport  Port=15
  In14 : Inport  Port=16
  In15 : Inport  Port=17
  In16 : Inport  Port=18
  Delay1 : xbsIndex_r4/Delay  rst=off  infoeditControl=Selection of Reset will increase slice count due to use of real FFs and instead of SRLs  en=off  latency=1  dbl_ovrd=off  reg_retiming=on  block_type=delay
  Delay2 : xbsIndex_r4/Delay  rst=off  infoeditControl=Selection of Reset will increase slice count due to use of real FFs and instead of SRLs  en=off  latency=1  dbl_ovrd=off  reg_retiming=on  block_type=delay
  Delay3 : xbsIndex_r4/Delay  rst=off  infoeditControl=Selection of Reset will increase slice count due to use of real FFs and instead of SRLs  en=off  latency=1  dbl_ovrd=off  reg_retiming=on  block_type=delay
  Delay_sync : xbsIndex_r4/Delay  rst=off  infoeditControl=Selection of Reset will increase slice count due to use of real FFs and instead of SRLs  en=off  latency=4  dbl_ovrd=off  reg_retiming=on  block_type=delay
  Mux{11..14,21..24,31..34,41..44,51..54,61..64,71..74,81..84,91..94,101..104,111..114,121..124,131..134,141..144,151..154,161..164} (64 alike) : xbsIndex_r4/Mux  inputs=2  en=off  latency=1  precision=Full  arith_type=Unsigned  n_bits=16  bin_pt=14  quantization=Truncate  overflow=Wrap  dbl_ovrd=off  block_type=mux
  Slice1 : xbsIndex_r4/Slice  nbits=1  boolean_output=off  mode=Upper Bit Location + Width  bit1=-0  base1=MSB of Input  bit0=0  base0=LSB of Input  dbl_ovrd=off  block_type=slice
  Slice2 : xbsIndex_r4/Slice  nbits=1  boolean_output=off  mode=Upper Bit Location + Width  bit1=-1  base1=MSB of Input  bit0=0  base0=LSB of Input  dbl_ovrd=off  block_type=slice
  Slice3 : xbsIndex_r4/Slice  nbits=1  boolean_output=off  mode=Upper Bit Location + Width  bit1=-2  base1=MSB of Input  bit0=0  base0=LSB of Input  dbl_ovrd=off  block_type=slice
  Slice4 : xbsIndex_r4/Slice  nbits=1  boolean_output=off  mode=Upper Bit Location + Width  bit1=-3  base1=MSB of Input  bit0=0  base0=LSB of Input  dbl_ovrd=off  block_type=slice
  sync_out : Outport
  Out1 : Outport  Port=2
  Out2 : Outport  Port=3
  Out3 : Outport  Port=4
  Out4 : Outport  Port=5
  Out5 : Outport  Port=6
  Out6 : Outport  Port=7
  Out7 : Outport  Port=8
  Out8 : Outport  Port=9
  Out9 : Outport  Port=10
  Out10 : Outport  Port=11
  Out11 : Outport  Port=12
  Out12 : Outport  Port=13
  Out13 : Outport  Port=14
  Out14 : Outport  Port=15
  Out15 : Outport  Port=16
  Out16 : Outport  Port=17
  wires:
  sync_in/1 -> Delay_sync/1
  Delay_sync/1 -> sync_out/1
  sel/1 -> Slice1/1, Delay1/1
  Delay1/1 -> Delay2/1, Slice2/1
  Delay2/1 -> Delay3/1, Slice3/1
  Delay3/1 -> Slice4/1
  Slice1/1 -> Mux11/1, Mux21/1, Mux31/1, Mux41/1, Mux51/1, Mux61/1, Mux71/1, Mux81/1, Mux91/1, Mux101/1, Mux111/1, Mux121/1, Mux131/1, Mux141/1, Mux151/1, Mux161/1
  Slice2/1 -> Mux12/1, Mux22/1, Mux32/1, Mux42/1, Mux52/1, Mux62/1, Mux72/1, Mux82/1, Mux92/1, Mux102/1, Mux112/1, Mux122/1, Mux132/1, Mux142/1, Mux152/1, Mux162/1
  Slice3/1 -> Mux13/1, Mux23/1, Mux33/1, Mux43/1, Mux53/1, Mux63/1, Mux73/1, Mux83/1, Mux93/1, Mux103/1, Mux113/1, Mux123/1, Mux133/1, Mux143/1, Mux153/1, Mux163/1
  Slice4/1 -> Mux14/1, Mux24/1, Mux34/1, Mux44/1, Mux54/1, Mux64/1, Mux74/1, Mux84/1, Mux94/1, Mux104/1, Mux114/1, Mux124/1, Mux134/1, Mux144/1, Mux154/1, Mux164/1
  In1/1 -> Mux11/2, Mux91/3
  Mux14/1 -> Out1/1
  In2/1 -> Mux21/2, Mux101/3
  Mux24/1 -> Out2/1
  In3/1 -> Mux31/2, Mux111/3
  Mux34/1 -> Out3/1
  In4/1 -> Mux41/2, Mux121/3
  Mux44/1 -> Out4/1
  In5/1 -> Mux51/2, Mux131/3
  Mux54/1 -> Out5/1
  In6/1 -> Mux61/2, Mux141/3
  Mux64/1 -> Out6/1
  In7/1 -> Mux71/2, Mux151/3
  Mux74/1 -> Out7/1
  In8/1 -> Mux81/2, Mux161/3
  Mux84/1 -> Out8/1
  In9/1 -> Mux91/2, Mux11/3
  Mux94/1 -> Out9/1
  In10/1 -> Mux101/2, Mux21/3
  Mux104/1 -> Out10/1
  In11/1 -> Mux111/2, Mux31/3
  Mux114/1 -> Out11/1
  In12/1 -> Mux121/2, Mux41/3
  Mux124/1 -> Out12/1
  In13/1 -> Mux131/2, Mux51/3
  Mux134/1 -> Out13/1
  In14/1 -> Mux141/2, Mux61/3
  Mux144/1 -> Out14/1
  In15/1 -> Mux151/2, Mux71/3
  Mux154/1 -> Out15/1
  In16/1 -> Mux161/2, Mux81/3
  Mux164/1 -> Out16/1
  Mux11/1 -> Mux12/2, Mux132/3
  Mux12/1 -> Mux13/2, Mux153/3
  Mux13/1 -> Mux14/2, Mux164/3
  Mux21/1 -> Mux22/2, Mux142/3
  Mux22/1 -> Mux23/2, Mux163/3
  Mux23/1 -> Mux24/2, Mux14/3
  Mux31/1 -> Mux32/2, Mux152/3
  Mux32/1 -> Mux33/2, Mux13/3
  Mux33/1 -> Mux34/2, Mux24/3
  Mux41/1 -> Mux42/2, Mux162/3
  Mux42/1 -> Mux43/2, Mux23/3
  Mux43/1 -> Mux44/2, Mux34/3
  Mux51/1 -> Mux52/2, Mux12/3
  Mux52/1 -> Mux53/2, Mux33/3
  Mux53/1 -> Mux54/2, Mux44/3
  Mux61/1 -> Mux62/2, Mux22/3
  Mux62/1 -> Mux63/2, Mux43/3
  Mux63/1 -> Mux64/2, Mux54/3
  Mux71/1 -> Mux72/2, Mux32/3
  Mux72/1 -> Mux73/2, Mux53/3
  Mux73/1 -> Mux74/2, Mux64/3
  Mux81/1 -> Mux82/2, Mux42/3
  Mux82/1 -> Mux83/2, Mux63/3
  Mux83/1 -> Mux84/2, Mux74/3
  Mux91/1 -> Mux92/2, Mux52/3
  Mux92/1 -> Mux93/2, Mux73/3
  Mux93/1 -> Mux94/2, Mux84/3
  Mux101/1 -> Mux102/2, Mux62/3
  Mux102/1 -> Mux103/2, Mux83/3
  Mux103/1 -> Mux104/2, Mux94/3
  Mux111/1 -> Mux112/2, Mux72/3
  Mux112/1 -> Mux113/2, Mux93/3
  Mux113/1 -> Mux114/2, Mux104/3
  Mux121/1 -> Mux122/2, Mux82/3
  Mux122/1 -> Mux123/2, Mux103/3
  Mux123/1 -> Mux124/2, Mux114/3
  Mux131/1 -> Mux132/2, Mux92/3
  Mux132/1 -> Mux133/2, Mux113/3
  Mux133/1 -> Mux134/2, Mux124/3
  Mux141/1 -> Mux142/2, Mux102/3
  Mux142/1 -> Mux143/2, Mux123/3
  Mux143/1 -> Mux144/2, Mux134/3
  Mux151/1 -> Mux152/2, Mux112/3
  Mux152/1 -> Mux153/2, Mux133/3
  Mux153/1 -> Mux154/2, Mux144/3
  Mux161/1 -> Mux162/2, Mux122/3
  Mux162/1 -> Mux163/2, Mux143/3
  Mux163/1 -> Mux164/2, Mux154/3

== system testing/delay_wideband_prog0/delay_dp0 ==
  din : Inport
  delay : Inport  Port=2
  AddSub : xbsIndex_r4/AddSub  mode=Subtraction  use_carryin=off  use_carryout=off  en=off  latency=1  precision=User Defined  arith_type=Unsigned  n_bits=ram_bits  bin_pt=0  quantization=Truncate  overflow=Wrap  dbl_ovrd=off  use_behavioral_HDL=on  hw_selection=Fabric  pipelined=off  use_rpm=on  block_type=addsub
  Constant2 : xbsIndex_r4/Constant  const=1  gui_display_data_type=Fixed-point  arith_type=Boolean  n_bits=1  bin_pt=0  preci_type=Single  exp_width=8  frac_width=24  explicit_period=on  period=1  equ=P=C  opselect=C  inp2=PCIN>>17  opr=+  inp1=P  carry=CIN  dbl_ovrd=off  block_type=constant
  Constant4 : xbsIndex_r4/Constant  const=0  gui_display_data_type=Fixed-point  arith_type=Boolean  n_bits=1  bin_pt=0  preci_type=Single  exp_width=8  frac_width=24  explicit_period=on  period=1  equ=P=C  opselect=C  inp2=PCIN>>17  opr=+  inp1=P  carry=CIN  dbl_ovrd=off  block_type=constant
  Dual Port RAM : xbsIndex_r4/Dual Port RAM  depth=2^ram_bits  initVector=0  distributed_mem=Block RAM  init_a=0  init_b=0  rst_a=off  rst_b=off  en_a=off  en_b=off  latency=bram_latency  write_mode_A=Read After Write  write_mode_B=Read Before Write  dbl_ovrd=off  optimize=Area  block_type=dpram
  Terminator : Terminator
  wr_addr : xbsIndex_r4/Counter  cnt_type=Free Running  cnt_to=Inf  operation=Up  start_count=0  cnt_by_val=1  arith_type=Unsigned  n_bits=ram_bits  bin_pt=0  load_pin=off  rst=off  en=off  explicit_period=on  period=1  dbl_ovrd=off  use_behavioral_HDL=on  implementation=Fabric  use_rpm=on  block_type=counter
  dout : Outport
  wires:
  delay/1 -> AddSub/2
  wr_addr/1 -> AddSub/1, Dual Port RAM/1
  din/1 -> Dual Port RAM/2, Dual Port RAM/5
  AddSub/1 -> Dual Port RAM/4
  Constant2/1 -> Dual Port RAM/3
  Constant4/1 -> Dual Port RAM/6
  Dual Port RAM/1 -> Terminator/1
  Dual Port RAM/2 -> dout/1
